simulink model "balloon_sim_temp"  (R2023b)
settings: Solver=ode3  StartTime=0.0  StopTime=600  FixedStep=0.01  RelTol=1e-3
settings Model: Creator=jerome  LastModifiedBy=jerome
settings ModelReferenceCC: EnableRefExpFcnMdlSchedulingChecks=on

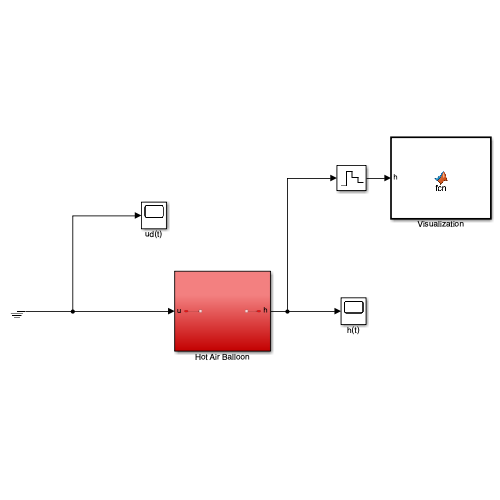
[thumbnail: Simulink's stored preview of the top-level diagram]
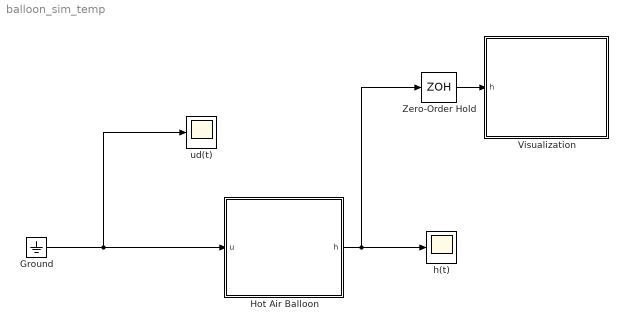
== system balloon_sim_temp ==
  Ground : Ground
  Hot Air Balloon : Subsystem
  Visualization : MATLAB Function  TreatAsAtomicUnit=on
  Zero-Order Hold : ZeroOrderHold  SampleTime=2
  h(t) : Scope
  ud(t) : Scope
  wires:
  Ground/1 -> ud(t)/1, Hot Air Balloon/1(u)
  Hot Air Balloon/1(h) -> Zero-Order Hold/1, h(t)/1
  Zero-Order Hold/1 -> Visualization/1(h)

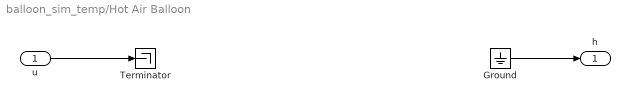
== system balloon_sim_temp/Hot Air Balloon ==
  u : Inport
  Ground : Ground
  Terminator : Terminator
  h : Outport
  wires:
  Ground/1 -> h/1
  u/1 -> Terminator/1

== matlab function balloon_sim_temp/Visualization ==
  data: h input
function fcn(h)

sf = 2.5; % scale factor
% balloon
    Xballoon = sf*[ 0 ; 0.6 ; 2.2 ; 3 ; 3 ; 2.2 ; 1.2 ; 0 ; -1.2 ; -2.2 ; -3 ; -3 ; -2.2 ; -0.6 ];
    Yballoon = sf*[ 1.2; 2; 3 ; 4 ; 5 ; 6; 6.4 ; 6.6 ; 6.4 ; 6 ; 5 ; 4 ; 3 ; 2 ]; 

% basket
    Xbasket = sf*[ 0.6 ; 0.6 ; -0.6 ; -0.6 ];
    Ybasket = sf*[ 0 ; 0.7 ; 0.7 ; 0 ];
    
% cables
    Xcable1 = sf*[ 0.6 ; 0.6 ];
    Ycable1 = sf*[ 0.7 ; 2 ];
    Xcable2 = sf*[ -0.6 ; -0.6 ];
    Ycable2 = sf*[ 0.7 ; 2 ];

    

% calculate graphical position of balloon
      PosXballoon = Xballoon;
      PosYballoon = Yballoon + h;

      PosXbasket = Xbasket;
      PosYbasket = Ybasket + h;

      PosXcable1 = Xcable1;
      PosYcable1 = Ycable1 + h;
      PosXcable2 = Xcable2;
      PosYcable2 = Ycable2 + h;

% to be able to use 'fill' even though the function is not supported for code generation
% see https://se.mathworks.com/help/simulink/slref/coder.extrinsic.html
coder.extrinsic('fill'); 

% draw the balloon
fill(PosXballoon,PosYballoon,'y');
hold on
brwn = [200 100 16]/256;
fill(PosXbasket,PosYbasket,brwn);
line(PosXcable1,PosYcable1,'Color','k','LineWidth',1);
line(PosXcable2,PosYcable2,'Color','k','LineWidth',1);
Xground = [-100;100];
Yground = [0;0];
Xgrass = [-100;-100;100;100];
Ygrass = [-20;0;0;-20];
line(Xground,Yground,'Color','k','LineWidth',3);
fill(Xgrass,Ygrass,'g');

hold off


axis([-60 60 -10 110]);
title('Open-loop control of a hot air balloon', 'FontSize',20);
axis square;
grid on;
lightBlue = [91, 207, 244] / 255;
set(gca,'Color',lightBlue);

drawnow;
